simulink model "lab6_4"  (R2022a)
settings: Solver=VariableStepAuto  StartTime=0.0  StopTime=10.0  RelTol=1e-3
undefined symbols (not defined in the file): Dopen, Nopen, t1, t2
settings Model: Creator=Egor  LastModifiedBy=Egor

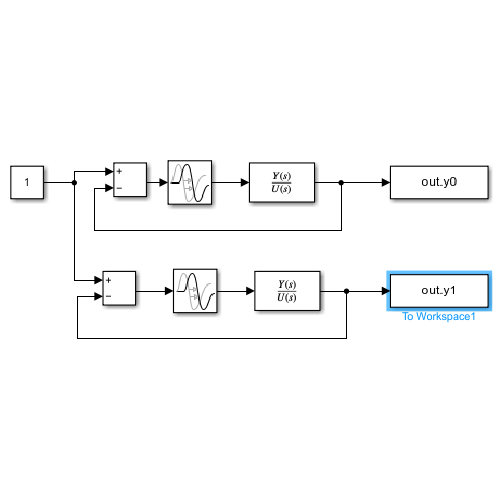
[thumbnail: Simulink's stored preview of the top-level diagram]
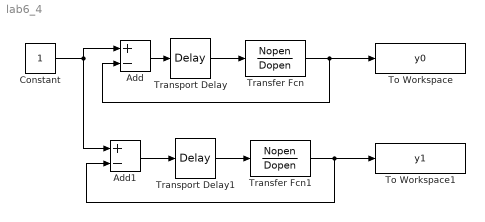
== system lab6_4 ==
  Add : Sum  Inputs=+-
  Add1 : Sum  Inputs=+-
  Constant : Constant
  To Workspace : ToWorkspace  VariableName=y0  SaveFormat=Timeseries  SampleTime=-1
  To Workspace1 : ToWorkspace  VariableName=y1  SaveFormat=Timeseries  SampleTime=-1
  Transfer Fcn : TransferFcn  Numerator=Nopen  Denominator=Dopen
  Transfer Fcn1 : TransferFcn  Numerator=Nopen  Denominator=Dopen
  Transport Delay : TransportDelay  DelayTime=t1
  Transport Delay1 : TransportDelay  DelayTime=t2
  wires:
  Add/1 -> Transport Delay/1
  Constant/1 -> Add1/1, Add/1
  Add1/1 -> Transport Delay1/1
  Transport Delay/1 -> Transfer Fcn/1
  Transport Delay1/1 -> Transfer Fcn1/1
  Transfer Fcn1/1 -> To Workspace1/1, Add1/2
  Transfer Fcn/1 -> Add/2, To Workspace/1
